simulink model "autosar_swc_fcncalls"  (R2022b)
settings: Solver=FixedStepDiscrete  StartTime=0.0  StopTime=10.0  FixedStep=1  RelTol=1e-3
settings Model: ModifiedByFormat=The MathWorks Inc.  Creator=The MathWorks, Inc.  LastModifiedBy=The MathWorks Inc.
settings SolverCC: AlgebraicLoopSolver=TrustRegion  MinimalZcImpactIntegration=on  MaxZcPerStep=1
settings DataIOCC: LimitDataPoints=on  SaveFormat=Array  SaveOutput=off  SaveTime=off  ReturnWorkspaceOutputs=off  SignalLoggingName=sigsOut
settings OptimizationCC: DefaultParameterBehavior=Inlined  UseDivisionForNetSlopeComputation=on  InlineInvariantSignals=on  EnhancedBackFolding=on  ExpressionDepthLimit=2147483647  StateBitsets=on  DataBitsets=on  ZeroExternalMemoryAtStartup=off  NoFixptDivByZeroProtection=on  EfficientFloat2IntCast=on  LifeSpan=1  EfficientTunableParamExpr=on
settings DebuggingCC: CheckExecutionContextPreStartOutputMsg=on  FcnCallInpInsideContextMsg=warning  AllowSymbolicDim=off  StateNameClashWarn=warning  PregeneratedLibrarySubsystemCodeDiagnostic=none  StrictBusMsg=ErrorOnBusTreatedAsVector  SFUnexpectedBacktrackingDiag=warning  SFNoUnconditionalDefaultTransitionDiag=warning  SFExecutionAtInitializationDiag=none  SFMachineParentedDataDiag=warning  ArithmeticOperatorsInVariantConditions=warning
settings HardwareCC: TargetHWDeviceType=Generic->32-bit Embedded Processor
settings ModelReferenceCC: UpdateModelReferenceTargets=IfOutOfDate  EnableRefExpFcnMdlSchedulingChecks=on  PropagateSignalLabelsOutOfModel=off
settings SFSimCC: SimUseLocalCustomCode=off  MATLABDynamicMemAlloc=off  CustomCodeUndefinedFunction=UseInterfaceOnly
settings RTWCC: Description=AUTOSAR  SystemTargetFile=autosar.tlc  TLCOptions=-p0 -aWarnNonSaturatedBlocks=0  GenCodeOnly=on  TemplateMakefile=ert_default_tmf  GenerateReport=on  RTWVerbose=off  RTWUseLocalCustomCode=off  IncludeHyperlinkInReport=on  LaunchReport=on  GenerateTraceInfo=on  GenerateTraceReport=on  GenerateTraceReportSl=on  GenerateTraceReportSf=on  GenerateTraceReportEml=on  GenerateCodeMetricsReport=on  DLArmComputeVersion=19.05
settings CodeAppCC: ForceParamTrailComments=on  IgnoreCustomStorageClasses=off  SimulinkDataObjDesc=on  CustomSymbolStrGlobalVar=rt$N$M  CustomSymbolStrType=$N$M  CustomSymbolStrFcn=$N$M$F  CustomSymbolStrModelFcn=$N  CustomSymbolStrMacro=$N$M  InsertBlockDesc=on  StateflowObjectComments=on
settings STFCustomTargetCC: UtilityFuncGeneration=Shared location  ParMdlRefBuildCompliant=on  CompOptLevelCompliant=on  IncludeMdlTerminateFcn=off  CombineOutputUpdateFcns=on  SuppressErrorStatus=on  ERTCustomFileBanners=on  SupportNonFinite=off  SupportComplex=off  SupportContinuousTime=off  SupportNonInlinedSFcns=off  RemoveResetFunc=on  MATLABClassNameForMDSCustomization=Simulink.SoftwareTarget.ERTCustomization  CPPClassGenCompliant=on  AutosarCompliant=on  UseToolchainInfoCompliant=on  LookupTableObjectStructAxisOrder=2,1,3,4,...  LUTObjectStructOrderEvenSpacing=Size,Table,Breakpoints  SystemTargetFile=autosar.tlc
settings ERTTargetCC: UtilityFuncGeneration=Shared location  MultiwordLength=2048  ConcurrentExecutionCompliant=off  IncludeMdlTerminateFcn=off  SuppressErrorStatus=on  SupportNonFinite=off  SupportComplex=off  ModelStepFunctionPrototypeControlCompliant=off  AutosarCompliant=on  LookupTableObjectStructAxisOrder=2,1,3,4,...  LUTObjectStructOrderEvenSpacing=Size,Table,Breakpoints  InlinedParameterPlacement=NonHierarchical  ERTCustomFileTemplate=example_file_process.tlc  ConvertIfToSwitch=off  SuppressUnreachableDefaultCases=off
settings ConfigComp: CovMetricSettings=dw  CovSaveCumulativeToWorkspaceVar=on  CovSaveSingleToWorkspaceVar=on  CovExternalEMLEnable=off  CovSFcnEnable=off

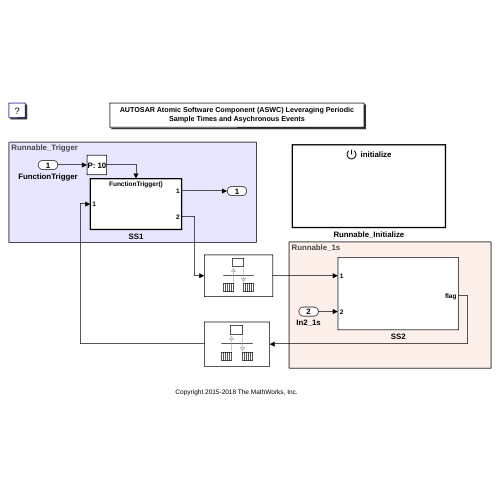
[thumbnail: Simulink's stored preview of the top-level diagram]
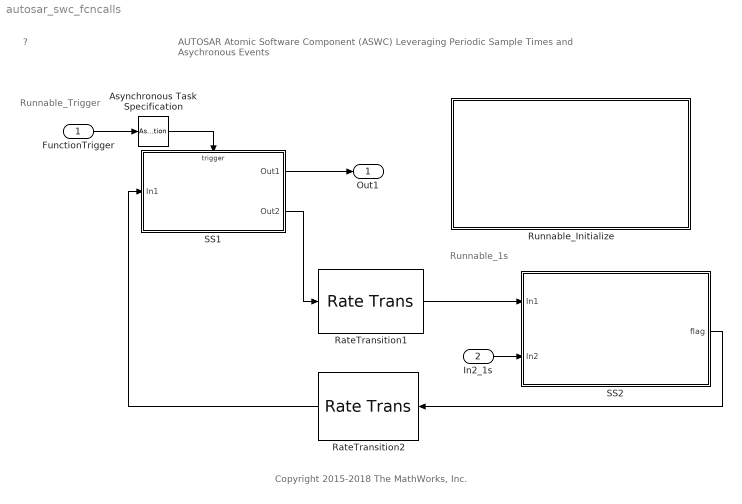
== system autosar_swc_fcncalls ==
  note: Runnable_1s
  note: Runnable_Trigger
  note: Copyright 2015-2018 The MathWorks, Inc.
  note: ?
  note: AUTOSAR Atomic Software Component (ASWC) Leveraging Periodic Sample Times and Asychronous Events
  FunctionTrigger : Inport  OutputFunctionCall=on
  In2_1s : Inport  Port=2  OutDataTypeStr=boolean  PortDimensions=1  SampleTime=1
  Asynchronous Task Specification : AsynchronousTaskSpecification
  RateTransition1 : RateTransition  Deterministic=off
  RateTransition2 : RateTransition  Deterministic=off
  Runnable_Initialize : Subsystem  TreatAsAtomicUnit=on
  SS1 : Subsystem
  SS2 : Subsystem
      settings: RTWSystemCode=Nonreusable function  RTWFcnNameOpts=Use subsystem name  RTWFileNameOpts=Use subsystem name
  Out1 : Outport  VectorParamsAs1DForOutWhenUnconnected=off
  wires:
  FunctionTrigger/1 -> Asynchronous Task Specification/1
  Asynchronous Task Specification/1 -> SS1/Trigger
  In2_1s/1 -> SS2/2(In2)
  RateTransition1/1 -> SS2/1(In1)
  SS2/1(flag) -> RateTransition2/1
  RateTransition2/1 -> SS1/1(In1)
  SS1/1(Out1) -> Out1/1
  SS1/2(Out2) -> RateTransition1/1

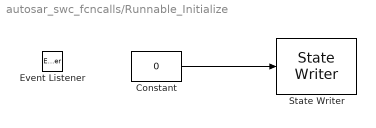
== system autosar_swc_fcncalls/Runnable_Initialize ==
  Constant : Constant  DisableCoverage=on  Value=0  OutDataTypeStr=boolean
  Event Listener : EventListener  DisableCoverage=on  EventName=reset
  State Writer : StateWriter  DisableCoverage=on  StateOwnerBlock=../../SS2/Unit Delay1
  wires:
  Constant/1 -> State Writer/1

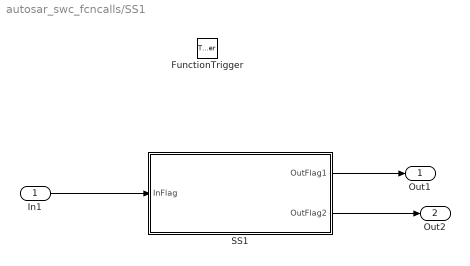
== system autosar_swc_fcncalls/SS1 ==
  In1 : Inport
  FunctionTrigger : TriggerPort  TriggerType=function-call  VariantControl=Variant  PortDimensions=1
  SS1 : Stateflow chart  TreatAsAtomicUnit=on
  Out1 : Outport  VectorParamsAs1DForOutWhenUnconnected=off
  Out2 : Outport  Port=2  VectorParamsAs1DForOutWhenUnconnected=off
  wires:
  SS1/2(OutFlag2) -> Out2/1
  In1/1 -> SS1/1(InFlag)
  SS1/1(OutFlag1) -> Out1/1

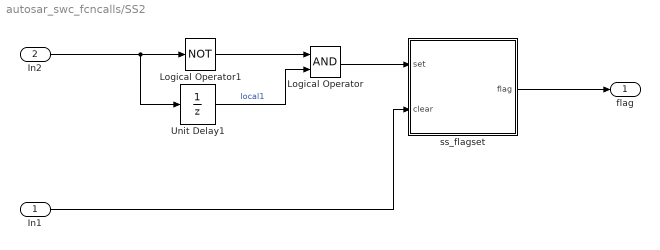
== system autosar_swc_fcncalls/SS2 ==
  In1 : Inport  PortDimensions=1  SampleTime=1
  In2 : Inport  Port=2  PortDimensions=1
  Logical Operator : Logic
  Logical Operator1 : Logic  Operator=NOT
  Unit Delay1 : UnitDelay  SampleTime=-1  HasFrameUpgradeWarning=on
  ss_flagset : Subsystem
  flag : Outport  VectorParamsAs1DForOutWhenUnconnected=off
  wires:
  Unit Delay1/1 -> Logical Operator/2  "local1"
  In2/1 -> Unit Delay1/1, Logical Operator1/1
  Logical Operator1/1 -> Logical Operator/1
  Logical Operator/1 -> ss_flagset/1(set)
  ss_flagset/1(flag) -> flag/1
  In1/1 -> ss_flagset/2(clear)

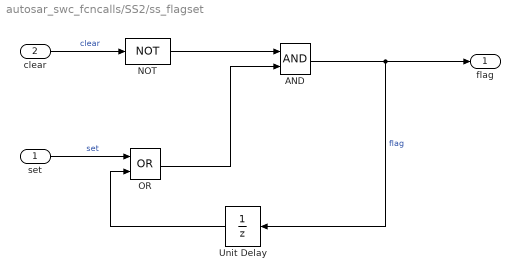
== system autosar_swc_fcncalls/SS2/ss_flagset ==
  set : Inport  OutDataTypeStr=boolean
  clear : Inport  Port=2  OutDataTypeStr=boolean
  AND : Logic  AllPortsSameDT=off  OutDataTypeStr=boolean
  NOT : Logic  Operator=NOT  AllPortsSameDT=off  OutDataTypeStr=boolean
  OR : Logic  Operator=OR  AllPortsSameDT=off  OutDataTypeStr=boolean
  Unit Delay : UnitDelay  SampleTime=-1  HasFrameUpgradeWarning=on
  flag : Outport  VectorParamsAs1DForOutWhenUnconnected=off
  wires:
  set/1 -> OR/1  "set"
  Unit Delay/1 -> OR/2
  AND/1 -> Unit Delay/1, flag/1  "flag"
  clear/1 -> NOT/1  "clear"
  NOT/1 -> AND/1
  OR/1 -> AND/2

== stateflow chart autosar_swc_fcncalls/SS1/SS1 ==
  state CON1/
    entry:
    OutFlag1 = 0;
    OutFlag2 = 0;
  state CON2/
    entry:
    OutFlag1 = 1;
    OutFlag2 = 1;
  state CON3/
    entry:
    OutFlag1 = 0;
    OutFlag2 = 1;
  (default) -> CON1
  CON1 -> CON2 : [InFlag==1]
  CON2 -> CON1 [order 1] : [InFlag == 0]
  CON2 -> CON3 [order 2]
  CON3 -> CON1 : [InFlag == 0]
  data: OutFlag1 output boolean; OutFlag2 output boolean; InFlag input boolean
